simulink model "sgMdl_IO751_IO752_PROFINETMultiNode"  (R2024b)
settings: Solver=FixedStepAuto  StartTime=0.0  StopTime=inf  RelTol=1e-3  EnableMultiTasking=on
undefined symbols (not defined in the file): C, DiscIntNeverNeededParam, Ts
libraries: slrealtimeutilitieslib x80, speedgoatlib_IO752 x6, speedgoatlib_IO751 x3, simulink x2
(part 2 of 2)

== system sgMdl_IO751_IO752_PROFINETMultiNode/IO752-32 PROFINET Device Simulation/Device 2 SINAMICS/Scale3 ==
  In1 : Inport
  Byte Reversal 4 : slrealtimeutilitieslib/Byte Reversal  numInp=1
  Data Type Conversion1 : DataTypeConversion  OutDataTypeStr=double  SaturateOnIntegerOverflow=off  RndMeth=Floor
  Gain2 : Gain  Gain=1/hex2dec('4000')
  Gain3 : Gain  Gain=8000
  Out1 : Outport
  wires:
  In1/1 -> Byte Reversal 4/1
  Gain2/1 -> Out1/1
  Gain3/1 -> Gain2/1
  Byte Reversal 4/1 -> Data Type Conversion1/1
  Data Type Conversion1/1 -> Gain3/1

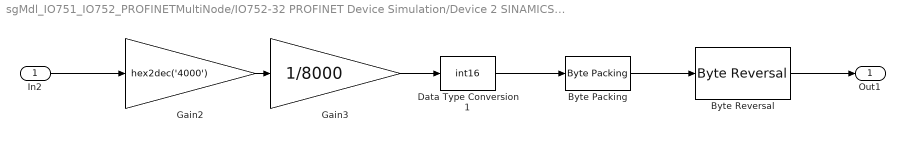
== system sgMdl_IO751_IO752_PROFINETMultiNode/IO752-32 PROFINET Device Simulation/Device 2 SINAMICS/Scale4 ==
  In2 : Inport  PortDimensions=1
  Byte Packing : slrealtimeutilitieslib/Byte Packing  MaskPackedDataType=uint16  MaskUnpackedDataTypes={'int16'}  MaskAlignment=1
  Byte Reversal : slrealtimeutilitieslib/Byte Reversal  numInp=1
  Data Type Conversion1 : DataTypeConversion  OutDataTypeStr=int16  SaturateOnIntegerOverflow=off  RndMeth=Floor
  Gain2 : Gain  Gain=hex2dec('4000')
  Gain3 : Gain  Gain=1/8000
  Out1 : Outport
  wires:
  In2/1 -> Gain2/1
  Byte Packing/1 -> Byte Reversal/1
  Data Type Conversion1/1 -> Byte Packing/1
  Byte Reversal/1 -> Out1/1
  Gain3/1 -> Data Type Conversion1/1
  Gain2/1 -> Gain3/1
